simulink model "check_tiredata_longitudinal"  (R2018b)
settings: configuration reference "Physics" (kept outside this file)
undefined symbols (not defined in the file or in its folder): Brakes, omega0_Wheels_radps
libraries: vehdynlibtire x1
settings Model: DataDictionary=check_tiredata.sldd  OrderedModelArguments=off  Creator=wischnewski  LastModifiedBy=ga25xiw

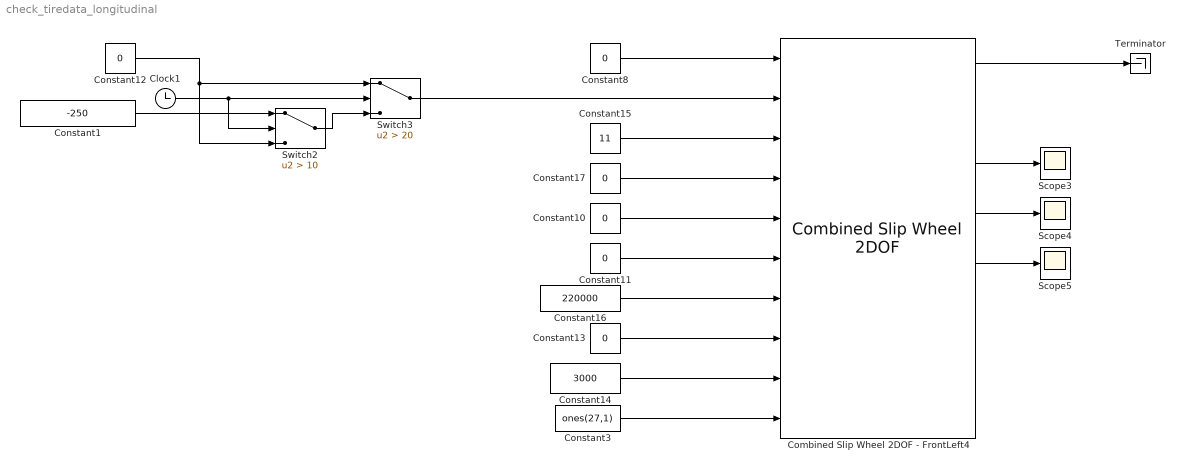
== system check_tiredata_longitudinal ==
  Clock1 : Clock
  Combined Slip Wheel 2DOF - FrontLeft4 : vehdynlibtire/Combined Slip Wheel 2DOF  BrakeType=Disc  mu_static=Brakes.mue_BrakePadsStaticFB (1)  mu_kinetic=Brakes.mue_BrakePadsKineticFB (1)  disk_abore=Brakes.d_BrakeBoreDiameterFB_m (1)  Rm=Brakes.r_BrakePadsMeanLeverRadiusFB_m (1)  num_pads=Brakes.n_BrakePadsNumberFB (1)  drum_abore=0.0508  drum_a=0.123  drum_c=0.212  drum_r=0.15  drum_theta1=0  drum_theta2=126  brake_p_bpt=[1 11.4736842105263 21.9473684210526 32.4210526315789 42.8947368421053 53.3684210526316 63.8421052631579 74.3157894736842 84.7894736842105 95.2631578947368 105.736842105263 116.210526315789 126.684210526316 137.157894736842 147.631578947368 158.105263157895 168.578947368421 179.052631578947 189.526315789474 200]  brake_n_bpt=[0 52.6315789473684 105.263157894737 157.894736842105 210.526315789474 263.157894736842 315.789473684211 368.421052631579 421.052631578947 473.684210526316 526.315789473684 578.947368421053 631.578947368421 684.210526315789 736.842105263158 789.473684210526 842.105263157895 894.736842105263 947.368421052632 1000]  f_brake_t=[43.4900602404453 42.5056030554862 41.5350898940194 40.5780454442085 39.6340111501808 38.7025443887544 37.7832176914519 36.8756180088306 35.9793460143796 35.0940154454303 34.2192524787115 33.3546951383474 32.4999927342521 31.6548053290159 30.8188032315107 29.991666515561 29.1730845621415 28.362755623661 27.5603864089927 26.765691687993;498.991217495636 487.695866636631 476.560505099801 465.579679307235 454.748127933653 444.060772460445 433.51270824929 423.099196101319 412.81565427025 402.657650900201 392.620896861006 382.701238955775 372.894653477208 363.197240090814 353.605216024701 344.114910546964 334.722759712992 325.425301366216 316.219170376863 307.10109410434;954.492374750826 932.886130217776 911.585920305583 890.581313170261 869.862244717126 849.419000532136 829.242198807128 809.322774193808 789.651962526121 770.221286354971 751.0225412433 732.047782773203 713.289314220164 694.739674852612 676.391628817892 658.238154578366 640.272434863842 622.48784710877 604.877954344734 587.436496520688;1409.99353200602 1378.07639379892 1346.61133551136 1315.58294703329 1284.9763615006 1254.77722860383 1224.97168936497 1195.5463522863 1166.48827078199 1137.78492180974 1109.42418562559 1081.39432659063 1053.68397496312 1026.28210961441 999.178041611083 972.361398609768 945.822110014692 919.550392851325 893.536738312604 867.771898937035;1865.49468926121 1823.26665738007 1781.63675071715 1740.58458089631 1700.09047828407 1660.13545667552 1620.7011799228 1581.76993037878 1543.32457903786 1505.34855726451 1467.82583000789 1430.74087040806 1394.07863570608 1357.82454437621 1321.96445440427 1286.48464264117 1251.37178516554 1216.61293859388 1182.19552228048 1148.10730135338;2320.9958465164 2268.45692096121 2216.66216592293 2165.58621475934 2115.20459506754 2065.49368474721 2016.43067048064 1967.99350847127 1920.16088729373 1872.91219271928 1826.22747439018 1780.08741422549 1734.47329644903 1689.36697913801 1644.75086719747 1600.60788667257 1556.92146031639 1513.67548433643 1470.85430624835 1428.44270376973;2776.49700377159 2713.64718454235 2651.68758112871 2590.58784862237 2530.31871185102 2470.8519128189 2412.16016103848 2354.21708656376 2296.9971955496 2240.47582817405 2184.62911877248 2129.43395804292 2074.86795719199 2020.9094138998 1967.53727999066 1914.73113070398 1862.47113546724 1810.73803007899 1759.51309021622 1708.77810618608;3231.99816102678 3158.8374481235 3086.71299633449 3015.58948248539 2945.43282863449 2876.21014089059 2807.88965159632 2740.44066465625 2673.83350380547 2608.03946362882 2543.03076315477 2478.78050186034 2415.26261793494 2352.4518486616 2290.32369278385 2228.85437473538 2168.02081061809 2107.80057582154 2048.17187418409 1989.11350860242;3687.49931828197 3604.02771170464 3521.73841154027 3440.59111634842 3360.54694541796 3281.56836896228 3203.61914215416 3126.66424274874 3050.66981206134 2975.60309908359 2901.43240753707 2828.12704567777 2755.6572786779 2683.9942834234 2613.11010557704 2542.97761876678 2473.57048576894 2404.8631215641 2336.83065815196 2269.44891101877;4143.00047553716 4049.21797528579 3956.76382674606 3865.59275021144 3775.66106220143 3686.92659703397 3599.34863271199 3512.88782084123 3427.50612031721 3343.16673453836 3259.83405191936 3177.4735894952 3096.05193942085 3015.5367181852 2935.89651837023 2857.10086279818 2779.12016091979 2701.92566730665 2625.48944211983 2549.78431343512;4598.50163279235 4494.40823886693 4391.78924195184 4290.59438407447 4190.77517898491 4092.28482510566 3995.07812326983 3899.11139893372 3804.34242857308 3710.73036999313 3618.23569630166 3526.82013331263 3436.44660016381 3347.079152947 3258.68293116342 3171.22410682959 3084.66983607064 2998.98821304921 2914.1482260877 2830.11971585147;5054.00279004754 4939.59850244808 4826.81465715762 4715.59601793749 4605.88929576838 4497.64305317735 4390.80761382767 4285.3349770262 4181.17873682896 4078.2940054479 3976.63734068395 3876.16667713006 3776.84126090677 3678.62158770879 3581.46934395661 3485.34735086099 ...(+2764 chars)]  tireParamSet=vdynPassCar.mat  plySteer=off  turnslip=off  PRESMAX=1000000  PRESMIN=10000  FZMAX=20000  FZMIN=1  VXLOW=1  KPUMAX=1.5  KPUMIN=-1.5  ALPMAX=1.5708  ALPMIN=-1.5708  CAMMAX=0.3147  CAMMIN=-0.3147  LONGVL=11  omegao=omega0_Wheels_radps (1)  br=0.1  UNLOADED_RADIUS=0.317  NOMPRES=220000  FNOMIN=3000  WIDTH=0.295  MASS=57  IYY=2.0  GRAVITY=-9.81  zo=0  zdoto=0  BREFF=3e-8  DREFF=0  FREFF=0  Q_RE0=1  Q_V1=0  Q_V2=0  Q_FZ1=25.36  Q_FZ2=0  Q_FZ3=0  Q_FCX=0  Q_FCY=0  Q_FCY2=0  PFZ1=0  VERTICAL_STIFFNESS=240000  VERTICAL_DAMPING=100  LONGITUDINAL_STIFFNESS=480000  LATERAL_STIFFNESS=120000  PCFX1=0  PCFX2=0  PCFX3=0  PCFY1=0  PCFY2=0  PCFY3=0  Q_RA1=0  Q_RA2=0  Q_RB1=0  Q_RB2=0  PCX1=1.6442  PDX1=1.5315  PDX2=-0.042865  PDX3=0.1  PEX1=0.69637  PEX2=-0.16976  PEX3=0.02267  PEX4=-0.14313  PKX1=30.732  PKX2=0.27129  PKX3=0.12779  PHX1=0  PHX2=0  PVX1=0  PVX2=0  PPX1=0  PPX2=0  PPX3=0  PPX4=0  RBX1=17.409  RBX2=12.892  RBX3=0  RCX1=1.0968  REX1=0  REX2=0  RHX1=0.0012757  QSX1=-0.00083931  QSX2=2.1019  QSX3=-0.036019  QSX4=0  QSX5=0  QSX6=0  QSX7=0  QSX8=0  QSX9=0  QSX10=0  QSX11=0  QSX12=0  QSX13=0  QSX14=0  PPMX1=0  PCY1=1.5675  PDY1=1.286  PDY2=-0.093005  PDY3=0.1  PEY1=0.10679  PEY2=-1.2054  PEY3=0.048624  PEY4=-8.1214  PEY5=0  PKY1=-75.4754  PKY2=4.6534  PKY3=-0.59931  PKY4=2  PKY5=0  PKY6=0  PKY7=0  PHY1=0.0028301  PHY2=-0.00063745  PVY1=0.040667  PVY2=-0.019226  PVY3=-0.96889  PVY4=-0.41406  PPY1=0  PPY2=0  PPY3=0  PPY4=0  PPY5=0  RBY1=20.57  RBY2=-23.533  RBY3=0.0010504  RBY4=0  RCY1=1.0094  REY1=0  REY2=0  RHY1=-0.019642  RHY2=0  RVY1=0.15504  RVY2=0.027779  RVY3=27.548  RVY4=-29.67  RVY5=0.033819  RVY6=0  QSY1=0.01  QSY2=0  QSY3=0  QSY4=0  QSY5=0  QSY6=0  QSY7=1  QSY8=1  QBZ1=9.0352  QBZ2=6.2747  QBZ3=-0.49801  QBZ4=-2.2859  QBZ5=2.687  QBZ6=0  QBZ9=-13.4538  QBZ10=0  QCZ1=1.1112  QDZ1=0.075296  QDZ2=0.0035884  QDZ3=-1.9194  QDZ4=-1.9825  QDZ6=-0.0050047  QDZ7=0.011095  QDZ8=-0.65039  QDZ9=-0.059214  QDZ10=0  QDZ11=0  QEZ1=-9.0284  QEZ2=11.0045  QEZ3=-5.8712  QEZ4=0.2394  QEZ5=-15.9158  QHZ1=0.0069694  QHZ2=-0.00091253  QHZ3=-0.18162  QHZ4=0.22912  PPZ1=0  PPZ2=0  SSZ1=-0.01265  SSZ2=0.048488  SSZ3=2.4368  SSZ4=-1.0105  PDXP1=0  PDXP2=0  PDXP3=0  PKYP1=0  PDYP1=0  PDYP2=0  PDYP3=0  PDYP4=0  PHYP1=0  PHYP2=0  PHYP3=0  PHYP4=0  PECP1=0  PECP2=0  QDTP1=0  QCRP1=0  QCRP2=0  QBRP1=0  QDRP1=0  QDRP2=0  aMode=2
      settings: SourceProductName=Vehicle Dynamics Blockset  SourceProductBaseCode=VE
  Constant1 : Constant  Value=-250
  Constant{8,10..13,17} (6 alike) : Constant  Value=0
  Constant14 : Constant  Value=3000
  Constant15 : Constant  Value=11
  Constant16 : Constant  Value=220000
  Constant3 : Constant  Value=ones(27,1)
  Scope3 : Scope
  Scope4 : Scope
  Scope5 : Scope
  Switch2 : Switch  Criteria=u2 > Threshold  Threshold=10
  Switch3 : Switch  Criteria=u2 > Threshold  Threshold=20
  Terminator : Terminator
  wires:
  Constant17/1 -> Combined Slip Wheel 2DOF - FrontLeft4/4
  Constant15/1 -> Combined Slip Wheel 2DOF - FrontLeft4/3
  Constant10/1 -> Combined Slip Wheel 2DOF - FrontLeft4/5
  Constant11/1 -> Combined Slip Wheel 2DOF - FrontLeft4/6
  Constant16/1 -> Combined Slip Wheel 2DOF - FrontLeft4/7
  Constant13/1 -> Combined Slip Wheel 2DOF - FrontLeft4/8
  Constant14/1 -> Combined Slip Wheel 2DOF - FrontLeft4/9
  Constant8/1 -> Combined Slip Wheel 2DOF - FrontLeft4/1
  Combined Slip Wheel 2DOF - FrontLeft4/5 -> Scope5/1
  Combined Slip Wheel 2DOF - FrontLeft4/4 -> Scope4/1
  Combined Slip Wheel 2DOF - FrontLeft4/3 -> Scope3/1
  Combined Slip Wheel 2DOF - FrontLeft4/1 -> Terminator/1
  Switch2/1 -> Switch3/3
  Constant12/1 -> Switch2/3, Switch3/1
  Clock1/1 -> Switch3/2, Switch2/2
  Constant1/1 -> Switch2/1
  Switch3/1 -> Combined Slip Wheel 2DOF - FrontLeft4/2
  Constant3/1 -> Combined Slip Wheel 2DOF - FrontLeft4/10
